simulink model "mpc_pendcartLTVMPC"  (R2023a)
settings: Solver=VariableStepAuto  StartTime=0.0  StopTime=20  MaxStep=1e-3  RelTol=1e-3  EnableMultiTasking=on
values from neighbouring files (symbols this model uses):
  PredictionHorizon = 60    [TimeVaryingMPCControlOfPendulum1.m]
  Ts = 0.01    [TimeVaryingMPCControlOfPendulum1.m]
  u0 = zeros(1,1)    [TimeVaryingMPCControlOfPendulum1.m]
libraries: mpclib x1, SignalEditorBlockLib x1
settings Model: Creator=The MathWorks, Inc.  LastModifiedBy=The MathWorks, Inc.
settings SolverCC: AlgebraicLoopSolver=LineSearch  MaxZcPerStep=1
settings DataIOCC: LimitDataPoints=on  SaveFormat=Array  SaveOutput=off  DSMLogging=off  SaveTime=off  ReturnWorkspaceOutputs=off
settings OptimizationCC: ReuseModelBlockBuffer=off  LifeSpan=inf
settings DebuggingCC: AlgebraicLoopMsg=none  UnderspecifiedInitializationDetection=Classic  MergeDetectMultiDrivingBlocksExec=none  SolverPrmCheckMsg=warning  UnconnectedInputMsg=warning  UnconnectedOutputMsg=warning  UnconnectedLineMsg=warning  AllowSymbolicDim=off  StateNameClashWarn=warning  SFUnexpectedBacktrackingDiag=warning  SFNoUnconditionalDefaultTransitionDiag=warning  SFExecutionAtInitializationDiag=none  ArithmeticOperatorsInVariantConditions=warning
settings HardwareCC: ProdBitPerPointer=32  ProdBitPerSizeT=32  ProdBitPerPtrDiffT=32  ProdLargestAtomicFloat=None  ProdIntDivRoundTo=Undefined  ProdEndianess=Unspecified  ProdWordSize=32  ProdHWDeviceType=32-bit Generic
settings ModelReferenceCC: EnableRefExpFcnMdlSchedulingChecks=on  PropagateSignalLabelsOutOfModel=off
settings SFSimCC: SimUseLocalCustomCode=off  CustomCodeUndefinedFunction=UseInterfaceOnly
settings RTWCC: RTWUseLocalCustomCode=off  DLArmComputeVersion=19.05
settings CodeAppCC: StateflowObjectComments=on
settings GRTTargetCC: TargetLangStandard=C89/C90 (ANSI)
settings ConfigComp: CovMetricSettings=dw  CovSaveCumulativeToWorkspaceVar=on  CovSaveSingleToWorkspaceVar=on  CovExternalEMLEnable=off  CovSFcnEnable=off
settings SimscapeCC: SimscapeNormalizeSystem=off  SimscapeNominalValues="[{\"value\":\"10\",\"unit\":\"V\"},{\"value\":\"1\",\"unit\":\"A\"},{\"value\":\"10\",\"unit\":\"N*m\"},{\"value\":\"10\",\"unit\":\"bar\"},{\"value\":\"100\",\"unit\":\"kJ/kg\"},{\"value\":\"1\",\"unit\":\"kW\"},{\"value\":\"300\",\"unit\":\"K\"},{\"value\":\"100\",\"unit\":\"cm^3/s\"},{\"value\":\"1\",\"unit\":\"kN\"},{\"value\":\"1\",\"unit\":\"g/cm^3\"},{\"value\":\"1\",\"unit\":\"l\"},{\"value\":\"1\",\"unit\":\"cm^2\"},{\"value\":\"60\",\"unit\":\"Hz\"}]"
settings ConfigurationSet: Description=SimMechanics 2G
settings ExplorerConfigSet: InternalSimMechanicsExplorerSettings="<ExplorerConfiguration><canonicalview>default</canonicalview><AnimationSetting><BasePlaybackSpeed>1.0</BasePlaybackSpeed><PlaybackSpeedFactor>1.0</PlaybackSpeedFactor></AnimationSetting><TilePanel><TileInfo><Tiles Columns=\"1\" Count=\"1\" Rows=\"1\"><Column Left=\"2\" Weight=\"1\"/><Column Left=\"1552\"/><Row Top=\"2\" Weight=\"1\"/><Row Top=\"932\"/><Tile Height=\"1\" Width=\"1\" X=\"0\" Y=\"0\"/></Tiles></TileInfo><SceneInfo><SceneViewer><BGColor><R>0.60000002384185791</R><G>0.60000002384185791</G><B>0.60000002384185791</B></BGColor><Camera><Position><X>0.027865189060748197</X><Y>-2.5719092456962986</Y><Z>0.23157896538506753</Z></Position><Center><X>0.62659712312732463</X><Y>-0.46110119691712204</Y><Z>0.22087365386473376</Z></Center><Up><X>-0.0079438354874226333</X><Y>0.0073246425924307582</Y><Z>0.99994162084025784</Z></Up><Left>-0.24533778208815546</Left><Right>0.24533778208815546</Right><Bottom>-0.79734779727023208</Bottom><Top>0.79734779727023208</Top></Camera></SceneViewer></SceneInfo></TilePanel></ExplorerConfiguration>"

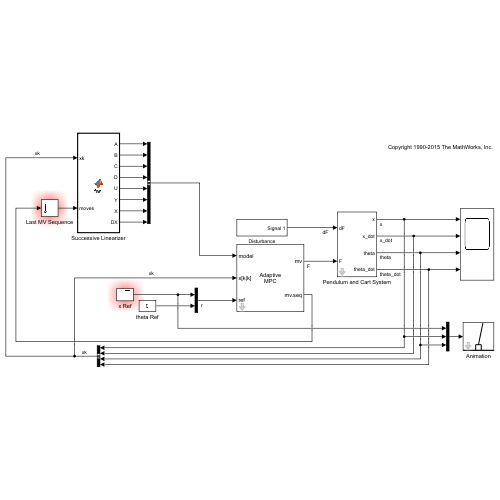
[thumbnail: Simulink's stored preview of the top-level diagram]
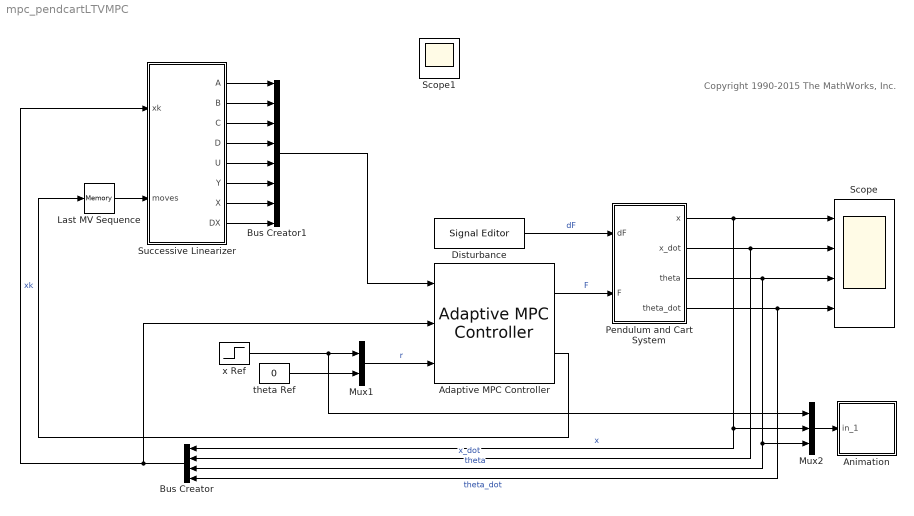
== system mpc_pendcartLTVMPC ==
  note: Copyright 1990-2015 The MathWorks, Inc.
  Adaptive MPC Controller : mpclib/Adaptive MPC Controller  SCDEnableBlockLinearizationSpecification=on  mpcobj=mpcobj  enable_value=0  updateMPCinCallerWorkspace=on  md_inport=off  mv_inport=off  uref_inport=off  return_cost=off  return_mvseq=on  return_qpstatus=off  return_xseq=off  return_state=off  return_ovseq=off  state_inport=on  isltv_plant=on  umin_inport=off  umax_inport=off  ymin_inport=off  ymax_inport=off  cc_inport=off  ywt_inport=off  uwt_inport=off  duwt_inport=off  rhoeps_inport=off  pm_inport=off  MaximumP=10  HorizonChoice=FixedHorizon  BlockDataType=double  SampleTimeInherited=off  switch_inport=off
  Animation : Subsystem  mask(Pendulum plot){RefBlock=x Ref}
      mask prompts: RefBlock "Cart Reference Signal Block Name:"
      mask help: Pendulum plot
      mask Help: Pendulum animation function using Handle graphics.
      mask Display: plot([-10 10],[0 0],[-2 -2 2 2],[0 1 1 0],[0 3],[1 5])
  Bus Creator : BusCreator  Inputs=4
  Bus Creator1 : BusCreator  Inputs=8
  Disturbance : SignalEditorBlockLib/Signal Editor  FileName=pendulumDisturbanceLTV.mat  ActiveScenario=Group_1  ActiveSignal=Signal 1  IsBus=off  OutputBusObjectStr=Bus: BusObject  SampleTime=0  OutputAfterFinalValue=Extrapolation  Unit=inherit  PreserveSignalName=on  ApplySigPropsToAllScenarios=on
  Last MV Sequence : Memory  InitialCondition=u0  InheritSampleTime=on
  Mux1 : Mux  Inputs=2
  Mux2 : Mux  Inputs=3
  Pendulum and Cart System : Subsystem  mask{mCartPara=1, mPendPara=1, gPara=9.81, LPara=0.5, KdPara=10}
      mask prompts: mCartPara "Mass of Cart"; mPendPara "Mass of Pendulum"; gPara "Gravity"; LPara "Length of Pendulum"; KdPara "Friction coefficient of Cart"
      mask help: Pendulum and Cart System
      mask init:
      | mCart = str2double(get_param(gcb,'mCartPara'));
      | mPend = str2double(get_param(gcb,'mPendPara'));
      | g = str2double(get_param(gcb,'gPara'));
      | L = str2double(get_param(gcb,'LPara'));
      | Kd = str2double(get_param(gcb,'KdPara'));
  Scope : Scope  NumInputPorts=4
  Successive Linearizer : MATLAB Function  TreatAsAtomicUnit=on
  theta Ref : Constant  Value=0
  x Ref : Step  After=20  SampleTime=Ts
  Scope1 : Scope
  wires:
  theta Ref/1 -> Mux1/2
  Pendulum and Cart System/4(theta_dot) -> Bus Creator/4, Scope/4  "theta_dot"
  Pendulum and Cart System/3(theta) -> Bus Creator/3, Mux2/3, Scope/3  "theta"
  Pendulum and Cart System/2(x_dot) -> Bus Creator/2, Scope/2  "x_dot"
  Pendulum and Cart System/1(x) -> Bus Creator/1, Mux2/2, Scope/1  "x"
  Disturbance/1 -> Pendulum and Cart System/1(dF)  "dF"
  Mux2/1 -> Animation/1(in_1)
  x Ref/1 -> Mux2/1, Mux1/1
  Bus Creator1/1 -> Adaptive MPC Controller/1
  Last MV Sequence/1 -> Successive Linearizer/2(moves)
  Mux1/1 -> Adaptive MPC Controller/3  "r"
  Successive Linearizer/1(A) -> Bus Creator1/1
  Successive Linearizer/2(B) -> Bus Creator1/2
  Successive Linearizer/3(C) -> Bus Creator1/3
  Successive Linearizer/4(D) -> Bus Creator1/4
  Successive Linearizer/5(U) -> Bus Creator1/5
  Successive Linearizer/6(Y) -> Bus Creator1/6
  Successive Linearizer/7(X) -> Bus Creator1/7
  Successive Linearizer/8(DX) -> Bus Creator1/8
  Bus Creator/1 -> Successive Linearizer/1(xk), Adaptive MPC Controller/2  "xk"
  Adaptive MPC Controller/1 -> Pendulum and Cart System/2(F)  "F"
  Adaptive MPC Controller/2 -> Last MV Sequence/1

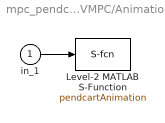
== system mpc_pendcartLTVMPC/Animation ==
  in_1 : Inport
  Level-2 MATLAB S-Function : M-S-Function  FunctionName=pendcartAnimation  Parameters=RefBlock
  wires:
  in_1/1 -> Level-2 MATLAB S-Function/1

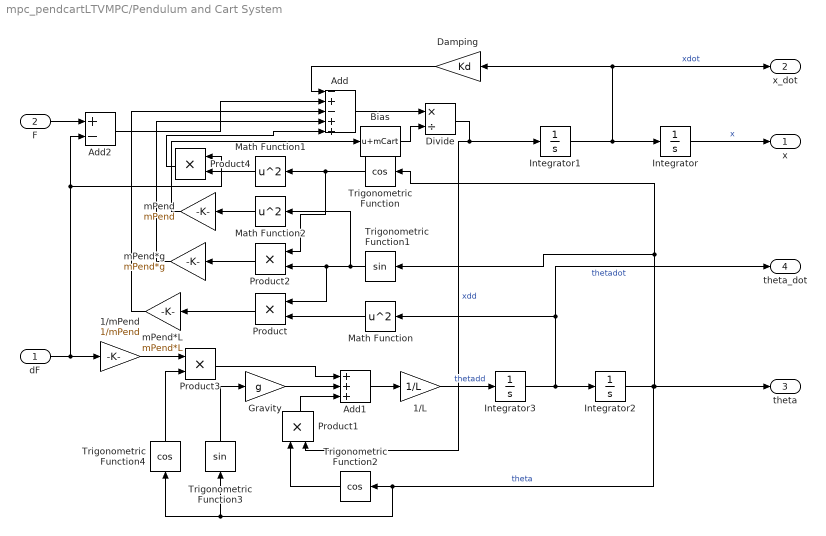
== system mpc_pendcartLTVMPC/Pendulum and Cart System ==
  dF : Inport
  F : Inport  Port=2
  1/L : Gain  Gain=1/L
  1/mPend : Gain  Gain=1/mPend
  Add : Sum  Inputs=-+-++
  Add1 : Sum  Inputs=+++
  Add2 : Sum  Inputs=+-
  Bias : Bias  Bias=mCart  SaturateOnIntegerOverflow=off
  Damping : Gain  Gain=Kd
  Divide : Product  Inputs=*/
  Gravity : Gain  Gain=g
  Integrator : Integrator  ContinuousStateAttributes='x'
  Integrator1 : Integrator  ContinuousStateAttributes='xdot'
  Integrator2 : Integrator  ContinuousStateAttributes='theta'
  Integrator3 : Integrator  ContinuousStateAttributes='thetadot'
  Math Function : Math  Operator=square  SignedPower=on
  Math Function1 : Math  Operator=square  SignedPower=on
  Math Function2 : Math  Operator=square  SignedPower=on
  Product{,1..4} (5 alike) : Product
  Trigonometric Function : Trigonometry  Operator=cos
  Trigonometric Function1 : Trigonometry
  Trigonometric Function2 : Trigonometry  Operator=cos
  Trigonometric Function3 : Trigonometry
  Trigonometric Function4 : Trigonometry  Operator=cos
  mPend : Gain  Gain=mPend
  mPend*L : Gain  Gain=mPend*L
  mPend*g : Gain  Gain=mPend*g
  x : Outport  VectorParamsAs1DForOutWhenUnconnected=off
  x_dot : Outport  Port=2  VectorParamsAs1DForOutWhenUnconnected=off
  theta : Outport  Port=3  VectorParamsAs1DForOutWhenUnconnected=off
  theta_dot : Outport  Port=4  VectorParamsAs1DForOutWhenUnconnected=off
  wires:
  mPend/1 -> Bias/1
  Bias/1 -> Divide/2
  Math Function2/1 -> mPend/1
  Product4/1 -> Add/5
  Math Function1/1 -> Product4/2
  mPend*g/1 -> Add/4
  Product1/1 -> Add1/3
  Math Function/1 -> Product/2
  1/L/1 -> Integrator3/1  "thetadd"
  dF/1 -> 1/mPend/1, Product4/1, Add2/2
  1/mPend/1 -> Product3/1
  Trigonometric Function4/1 -> Product3/2
  Damping/1 -> Add/1
  F/1 -> Add2/1
  Trigonometric Function3/1 -> Gravity/1
  Gravity/1 -> Add1/2
  Trigonometric Function/1 -> Math Function1/1, Product2/1
  Integrator3/1 -> Integrator2/1, Math Function/1, theta_dot/1  "thetadot"
  Integrator2/1 -> Trigonometric Function2/1, Trigonometric Function3/1, Trigonometric Function4/1, Trigonometric Function1/1, Trigonometric Function/1, theta/1  "theta"
  Product3/1 -> Add1/1
  Add/1 -> Divide/1
  Divide/1 -> Integrator1/1, Product1/2  "xdd"
  Trigonometric Function2/1 -> Product1/1
  Trigonometric Function1/1 -> Math Function2/1, Product/1, Product2/2
  Integrator/1 -> x/1  "x"
  Integrator1/1 -> Damping/1, x_dot/1, Integrator/1  "xdot"
  Product2/1 -> mPend*g/1
  Add1/1 -> 1/L/1
  Add2/1 -> Add/2
  mPend*L/1 -> Add/3
  Product/1 -> mPend*L/1

== matlab function mpc_pendcartLTVMPC/Successive Linearizer ==
  settings: updateMethod=DISCRETE  sampleTime=Ts
  data: xk input; moves input; A output; B output; C output; D output; U output; Y output; X output; DX output; Ts parameter; PredictionHorizon parameter
function [A,B,C,D,U,Y,X,DX] = fcn(xk,moves,Ts,PredictionHorizon)
% LTV MPC requires p+1 linearizations from k to k+p
Steps = PredictionHorizon + 1;
% Initialize outputs
A = zeros(4,4,Steps);
B = zeros(4,1,Steps);
C = zeros(2,4,Steps);
D = zeros(2,1,Steps);
U = zeros(1,1,Steps);
Y = zeros(2,1,Steps);
X = zeros(4,1,Steps);
DX = zeros(4,1,Steps);
% Obtain time varying linear models via successive linearization
for ct = 1:Steps
    % since we don't have u(k) ... u(k+p) at the time of linearization,
    % previous optimal sequence u(k-1) ... u(k+p-1) is used instead.
    if ct>length(moves)
        uk = moves(end);
    else
        uk = moves(ct);
    end
    % analytical linearization (continuous time)
    [DXk, yk, Ak, Bk0, Ck, Dk] = pendulumCT(xk, uk);
    % append dx offset 
    Bk = [Bk0 DXk];
    % convert A and B matrices from continuous time to discrete time
    [Ak, Bk] = adasblocks_utilDicretizeModel(Ak, Bk, Ts);
    % obtain matrices
    A(:,:,ct) = Ak;
    B(:,:,ct) = Bk(:,1);
    C(:,:,ct) = Ck([1 3],:);
    D(:,:,ct) = Dk([1 3],:);
    U(:,:,ct) = uk;
    Y(:,:,ct) = yk([1 3]);
    X(:,:,ct) = xk;
    DX(:,:,ct) = Bk(:,2);
    % next prediction step
    xk = pendulumDT(xk, uk, Ts);
end

function [A, B] = getDiscrete(a, b, Ts)
% Convert A, B to discrete time
A = expm(a*Ts);
nx = size(b,1);
n = 4;  % Number of points for Simpson's Rule, an even integer >= 2.
% Use Simpson's rule to compute integral(0,Ts){expm(a*s)*ds*b}
h = Ts/n;
Ai = eye(nx) + A;        % First and last terms;
Coef = 2;
for i = 1:n-1
    if Coef == 2
        Coef = 4;
    else
        Coef = 2;
    end
    Ai = Ai + Coef*expm(a*i*h);     % Intermediate terms
end
B = (h/3)*Ai*b;
